simulink model "Modelo_nolineal_5GDL_2021"  (R2021b)
settings: Solver=VariableStepAuto  StartTime=0.0  StopTime=5  FixedStep=T  RelTol=1e-3
values from neighbouring files (symbols this model uses):
  g = 9.81    [Control_5GDL_2021.m]
  Ixx = pod.mass.inertia(1,1)    [Control_5GDL_2021.m]
  Iyy = pod.mass.inertia(2,2)    [Control_5GDL_2021.m]
  Izz = pod.mass.inertia(3,3)    [Control_5GDL_2021.m]
  m = pod.mass.mass    [Control_5GDL_2021.m]
  theta0 = 0    [Control_5GDL_2021.m]
  x_g = pod.geometry.x_G    [Control_5GDL_2021.m]
  x_lev = pod.geometry.x_LEV    [Control_5GDL_2021.m]
  y_lev = pod.geometry.y_LEV    [Control_5GDL_2021.m]
  z_g = pod.geometry.z_G    [Control_5GDL_2021.m]
  z_ini = z_0+z_lev    [Control_5GDL_2021.m]
undefined symbols (not defined in the file or in its folder): k1, k2, k3, k4, l1, l2, l3, p1, p2
settings Model: Creator=EDMAOR  LastModifiedBy=emate
settings SolverCC: AlgebraicLoopSolver=TrustRegion
settings DebuggingCC: SFMachineParentedDataDiag=warning
settings SFSimCC: CustomCodeUndefinedFunction=UseInterfaceOnly

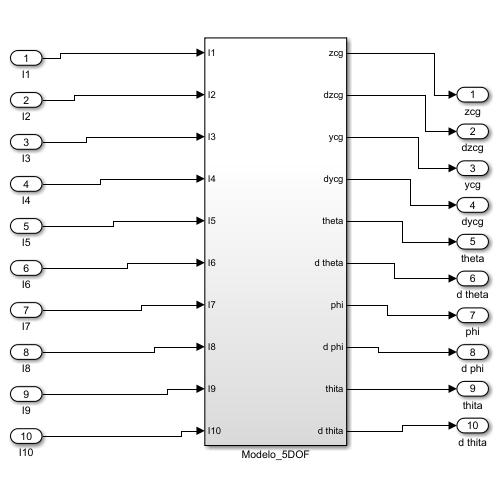
[thumbnail: Simulink's stored preview of the top-level diagram]
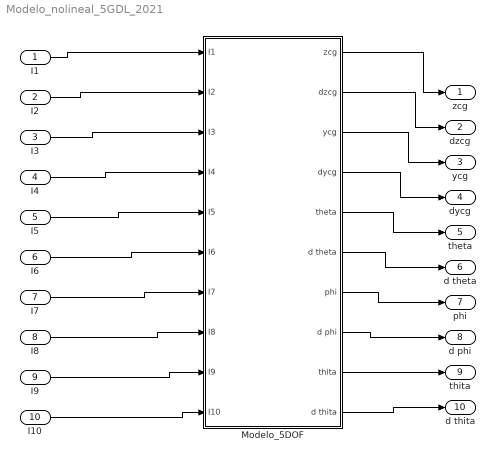
== system Modelo_nolineal_5GDL_2021 ==
  I1 : Inport
  I2 : Inport  Port=2
  I3 : Inport  Port=3
  I4 : Inport  Port=4
  I5 : Inport  Port=5
  I6 : Inport  Port=6
  I7 : Inport  Port=7
  I8 : Inport  Port=8
  I9 : Inport  Port=9
  I10 : Inport  Port=10
  Modelo_5DOF : Subsystem
  zcg : Outport  VectorParamsAs1DForOutWhenUnconnected=off
  dzcg : Outport  Port=2  VectorParamsAs1DForOutWhenUnconnected=off
  ycg : Outport  Port=3  VectorParamsAs1DForOutWhenUnconnected=off
  dycg : Outport  Port=4  VectorParamsAs1DForOutWhenUnconnected=off
  theta : Outport  Port=5  VectorParamsAs1DForOutWhenUnconnected=off
  d theta : Outport  Port=6  VectorParamsAs1DForOutWhenUnconnected=off
  phi : Outport  Port=7  VectorParamsAs1DForOutWhenUnconnected=off
  d phi : Outport  Port=8  VectorParamsAs1DForOutWhenUnconnected=off
  thita : Outport  Port=9  VectorParamsAs1DForOutWhenUnconnected=off
  d thita : Outport  Port=10  VectorParamsAs1DForOutWhenUnconnected=off
  wires:
  Modelo_5DOF/1(zcg) -> zcg/1
  I1/1 -> Modelo_5DOF/1(I1)
  I2/1 -> Modelo_5DOF/2(I2)
  I3/1 -> Modelo_5DOF/3(I3)
  I4/1 -> Modelo_5DOF/4(I4)
  I5/1 -> Modelo_5DOF/5(I5)
  I6/1 -> Modelo_5DOF/6(I6)
  Modelo_5DOF/2(dzcg) -> dzcg/1
  Modelo_5DOF/3(ycg) -> ycg/1
  Modelo_5DOF/4(dycg) -> dycg/1
  Modelo_5DOF/5(theta) -> theta/1
  Modelo_5DOF/6(d theta) -> d theta/1
  Modelo_5DOF/7(phi) -> phi/1
  Modelo_5DOF/8(d phi) -> d phi/1
  I7/1 -> Modelo_5DOF/7(I7)
  I8/1 -> Modelo_5DOF/8(I8)
  I9/1 -> Modelo_5DOF/9(I9)
  I10/1 -> Modelo_5DOF/10(I10)
  Modelo_5DOF/9(thita) -> thita/1
  Modelo_5DOF/10(d thita) -> d thita/1

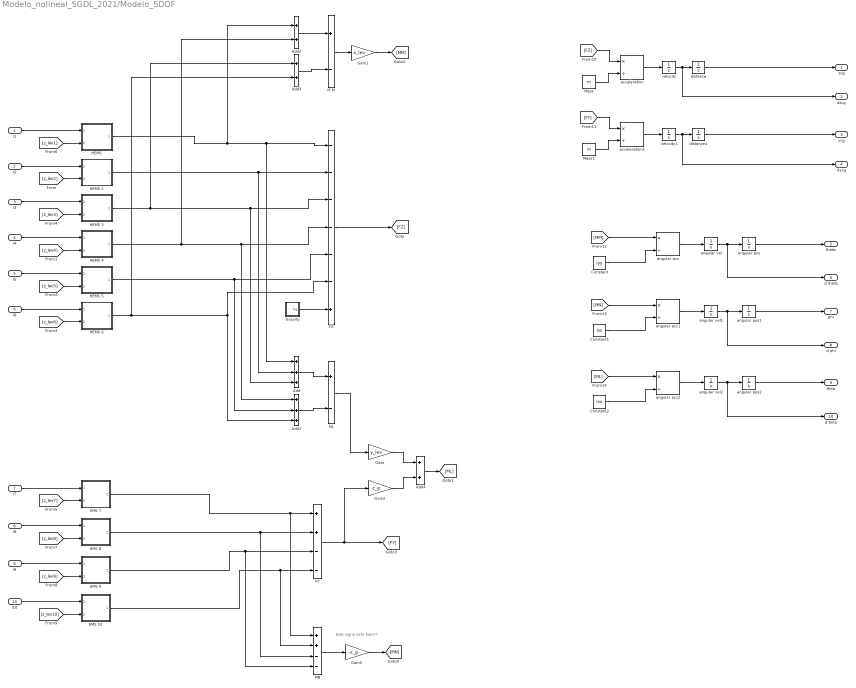
== system Modelo_nolineal_5GDL_2021/Modelo_5DOF ==
  note: Este signo esta bien??
  I1 : Inport
  I2 : Inport  Port=2
  I3 : Inport  Port=3
  I4 : Inport  Port=4
  I5 : Inport  Port=5
  I6 : Inport  Port=6
  I7 : Inport  Port=7
  I8 : Inport  Port=8
  I9 : Inport  Port=9
  I10 : Inport  Port=10
  Add : Sum  Inputs=+++
  Add1 : Sum  Inputs=+++
  Add2 : Sum
  Add3 : Sum
  Add4 : Sum
  Constant : Constant  Value=Iyy
  Constant1 : Constant  Value=Izz
  Constant2 : Constant  Value=Ixx
  EMS 10 : Subsystem
  EMS 7 : Subsystem
  EMS 8 : Subsystem
  EMS 9 : Subsystem
  FY : Sum  Inputs=++--
  FZ : Sum  Inputs=------+
  Gain : Gain  Gain=y_lev
  Gain1 : Gain  Gain=x_lev
  Gain2 : Gain  Gain=z_g
  Gain5 : Gain  Gain=-x_g
  Gravity : Subsystem
  "HEMS " : Subsystem
  HEMS 2 : Subsystem
  HEMS 3 : Subsystem
  HEMS 4 : Subsystem
  HEMS 5 : Subsystem
  HEMS 6 : Subsystem
  M M : Sum  Inputs=+-
  ML : Sum  Inputs=+-
  MN : Sum  Inputs=++--
  Mass : Constant  Value=m
  Mass1 : Constant  Value=m
  acceleration : Product  Inputs=*/
  acceleration1 : Product  Inputs=*/
  angular acc : Product  Inputs=*/
  angular acc1 : Product  Inputs=*/
  angular acc2 : Product  Inputs=*/
  angular pos : Integrator  InitialCondition=theta0
  angular pos1 : Integrator  InitialCondition=theta0
  angular pos2 : Integrator  InitialCondition=theta0
  angular vel : Integrator
  angular vel1 : Integrator
  angular vel2 : Integrator
  distance : Integrator  InitialCondition=z_ini
  distance1 : Integrator
  velocity : Integrator
  velocity1 : Integrator
  zcg : Outport  VectorParamsAs1DForOutWhenUnconnected=off
  dzcg : Outport  Port=2  VectorParamsAs1DForOutWhenUnconnected=off
  ycg : Outport  Port=3  VectorParamsAs1DForOutWhenUnconnected=off
  dycg : Outport  Port=4  VectorParamsAs1DForOutWhenUnconnected=off
  theta : Outport  Port=5  VectorParamsAs1DForOutWhenUnconnected=off
  d theta : Outport  Port=6  VectorParamsAs1DForOutWhenUnconnected=off
  phi : Outport  Port=7  VectorParamsAs1DForOutWhenUnconnected=off
  d phi : Outport  Port=8  VectorParamsAs1DForOutWhenUnconnected=off
  thita : Outport  Port=9  VectorParamsAs1DForOutWhenUnconnected=off
  d thita : Outport  Port=10  VectorParamsAs1DForOutWhenUnconnected=off
  wires:
  acceleration/1 -> velocity/1
  velocity/1 -> dzcg/1, distance/1
  distance/1 -> zcg/1
  I1/1 -> "HEMS "/1(current 1)
  I2/1 -> HEMS 2/1(current 2)
  I3/1 -> HEMS 3/1(current 3)
  "HEMS "/1(HEMS 1) -> Add/1, FZ/1, Add2/1
  HEMS 2/1(HEMS 2) -> Add/2, FZ/2
  HEMS 3/1(HEMS 3) -> Add/3, FZ/3, Add3/1
  Mass/1 -> acceleration/2
  [z_lev2] -> HEMS 2/2(distance 2)
  [z_lev3] -> HEMS 3/2(distance 3)
  [z_lev1] -> "HEMS "/2(distance 1)
  I4/1 -> HEMS 4/1(current 4)
  I5/1 -> HEMS 5/1(current 5)
  I6/1 -> HEMS 6/1(current 6)
  [z_lev4] -> HEMS 4/2(distance 4)
  [z_lev5] -> HEMS 5/2(distance 5)
  [z_lev6] -> HEMS 6/2(distance 6)
  HEMS 4/1(HEMS 4) -> Add1/1, FZ/4, Add2/2
  HEMS 5/1(HEMS 5) -> Add1/2, FZ/5
  HEMS 6/1(HEMS 6) -> Add1/3, FZ/6, Add3/2
  Gravity/1(Fg) -> FZ/7
  FZ/1 -> [FZ]
  ML/1 -> Gain/1
  Add1/1 -> ML/2
  Add/1 -> ML/1
  M M/1 -> Gain1/1
  Gain1/1 -> [MM]
  Add2/1 -> M M/1
  Add3/1 -> M M/2
  I7/1 -> EMS 7/1(current 7)
  [z_lev7] -> EMS 7/2(distance 7)
  I8/1 -> EMS 8/1(current 8)
  [z_lev8] -> EMS 8/2(distance 8)
  I9/1 -> EMS 9/1(current 9)
  [z_lev9] -> EMS 9/2(distance 9)
  I10/1 -> EMS 10/1(current 10)
  [z_lev10] -> EMS 10/2(distance 10)
  EMS 7/1(EMS 7) -> MN/1, FY/1
  EMS 8/1(EMS 8) -> MN/3, FY/2
  EMS 9/1(EMS 9) -> MN/4, FY/3
  EMS 10/1(EMS 10) -> MN/2, FY/4
  FY/1 -> [FY], Gain2/1
  Add4/1 -> [ML]
  Gain/1 -> Add4/1
  Gain2/1 -> Add4/2
  MN/1 -> Gain5/1
  Gain5/1 -> [MN]
  [FZ] -> acceleration/1
  [FY] -> acceleration1/1
  Mass1/1 -> acceleration1/2
  distance1/1 -> ycg/1
  velocity1/1 -> distance1/1, dycg/1
  acceleration1/1 -> velocity1/1
  angular vel/1 -> d theta/1, angular pos/1
  angular pos/1 -> theta/1
  angular acc/1 -> angular vel/1
  [MM] -> angular acc/1
  Constant/1 -> angular acc/2
  angular acc1/1 -> angular vel1/1
  Constant1/1 -> angular acc1/2
  angular vel1/1 -> d phi/1, angular pos1/1
  [MN] -> angular acc1/1
  angular pos1/1 -> phi/1
  angular pos2/1 -> thita/1
  [ML] -> angular acc2/1
  angular vel2/1 -> angular pos2/1, d thita/1
  Constant2/1 -> angular acc2/2
  angular acc2/1 -> angular vel2/1

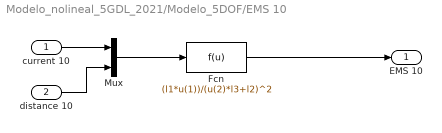
== system Modelo_nolineal_5GDL_2021/Modelo_5DOF/EMS 10 ==
  current 10 : Inport
  distance 10 : Inport  Port=2
  Fcn : Fcn  Expr=(l1*u(1))/(u(2)*l3+l2)^2
  Mux : Mux  Inputs=2
  EMS 10 : Outport  VectorParamsAs1DForOutWhenUnconnected=off
  wires:
  Fcn/1 -> EMS 10/1
  Mux/1 -> Fcn/1
  distance 10/1 -> Mux/2
  current 10/1 -> Mux/1

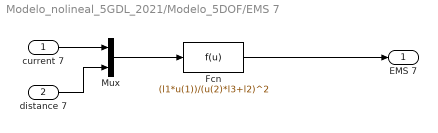
== system Modelo_nolineal_5GDL_2021/Modelo_5DOF/EMS 7 ==
  current 7 : Inport
  distance 7 : Inport  Port=2
  Fcn : Fcn  Expr=(l1*u(1))/(u(2)*l3+l2)^2
  Mux : Mux  Inputs=2
  EMS 7 : Outport  VectorParamsAs1DForOutWhenUnconnected=off
  wires:
  current 7/1 -> Mux/1
  distance 7/1 -> Mux/2
  Mux/1 -> Fcn/1
  Fcn/1 -> EMS 7/1

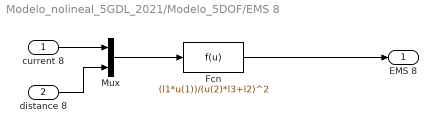
== system Modelo_nolineal_5GDL_2021/Modelo_5DOF/EMS 8 ==
  current 8 : Inport
  distance 8 : Inport  Port=2
  Fcn : Fcn  Expr=(l1*u(1))/(u(2)*l3+l2)^2
  Mux : Mux  Inputs=2
  EMS 8 : Outport  VectorParamsAs1DForOutWhenUnconnected=off
  wires:
  Fcn/1 -> EMS 8/1
  Mux/1 -> Fcn/1
  distance 8/1 -> Mux/2
  current 8/1 -> Mux/1

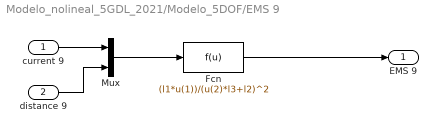
== system Modelo_nolineal_5GDL_2021/Modelo_5DOF/EMS 9 ==
  current 9 : Inport
  distance 9 : Inport  Port=2
  Fcn : Fcn  Expr=(l1*u(1))/(u(2)*l3+l2)^2
  Mux : Mux  Inputs=2
  EMS 9 : Outport  VectorParamsAs1DForOutWhenUnconnected=off
  wires:
  current 9/1 -> Mux/1
  distance 9/1 -> Mux/2
  Mux/1 -> Fcn/1
  Fcn/1 -> EMS 9/1

== system Modelo_nolineal_5GDL_2021/Modelo_5DOF/Gravity ==
  Fgrav : Subsystem
  Mass : Constant  Value=m
  gravity : Constant  Value=g
  Fg : Outport
  wires:
  Fgrav/1(Fg) -> Fg/1
  gravity/1 -> Fgrav/1(gravity)
  Mass/1 -> Fgrav/2(mass)

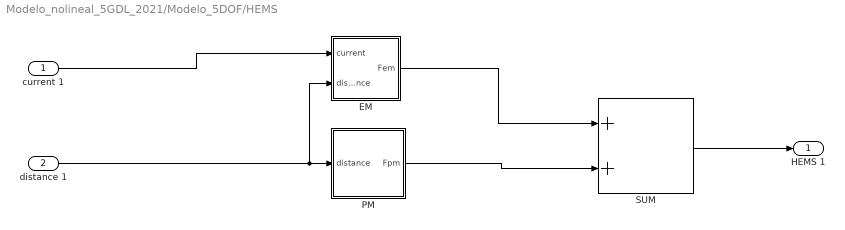
== system Modelo_nolineal_5GDL_2021/Modelo_5DOF/HEMS  ==
  current 1 : Inport
  distance 1 : Inport  Port=2
  EM : Subsystem
  PM : Subsystem
  SUM : Sum
  HEMS 1 : Outport  VectorParamsAs1DForOutWhenUnconnected=off
  wires:
  PM/1(Fpm) -> SUM/2
  distance 1/1 -> EM/2(distance), PM/1(distance)
  EM/1(Fem) -> SUM/1
  current 1/1 -> EM/1(current)
  SUM/1 -> HEMS 1/1

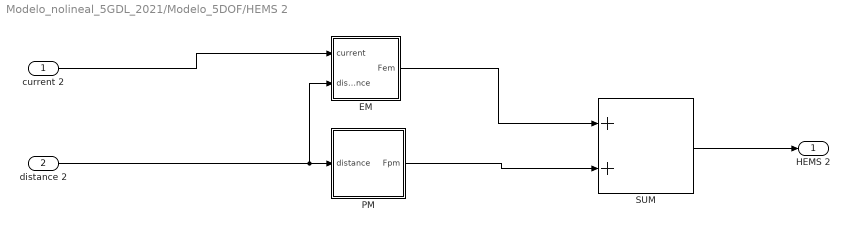
== system Modelo_nolineal_5GDL_2021/Modelo_5DOF/HEMS 2 ==
  current 2 : Inport
  distance 2 : Inport  Port=2
  EM : Subsystem
  PM : Subsystem
  SUM : Sum
  HEMS 2 : Outport  VectorParamsAs1DForOutWhenUnconnected=off
  wires:
  SUM/1 -> HEMS 2/1
  current 2/1 -> EM/1(current)
  EM/1(Fem) -> SUM/1
  distance 2/1 -> PM/1(distance), EM/2(distance)
  PM/1(Fpm) -> SUM/2

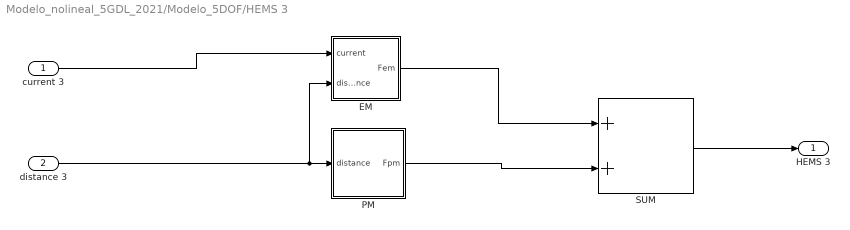
== system Modelo_nolineal_5GDL_2021/Modelo_5DOF/HEMS 3 ==
  current 3 : Inport
  distance 3 : Inport  Port=2
  EM : Subsystem
  PM : Subsystem
  SUM : Sum
  HEMS 3 : Outport  VectorParamsAs1DForOutWhenUnconnected=off
  wires:
  PM/1(Fpm) -> SUM/2
  distance 3/1 -> EM/2(distance), PM/1(distance)
  EM/1(Fem) -> SUM/1
  current 3/1 -> EM/1(current)
  SUM/1 -> HEMS 3/1

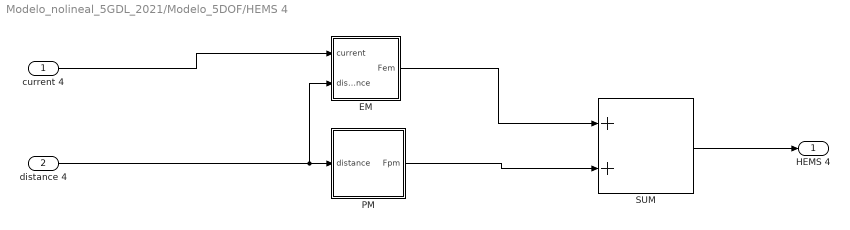
== system Modelo_nolineal_5GDL_2021/Modelo_5DOF/HEMS 4 ==
  current 4 : Inport
  distance 4 : Inport  Port=2
  EM : Subsystem
  PM : Subsystem
  SUM : Sum
  HEMS 4 : Outport  VectorParamsAs1DForOutWhenUnconnected=off
  wires:
  SUM/1 -> HEMS 4/1
  current 4/1 -> EM/1(current)
  EM/1(Fem) -> SUM/1
  distance 4/1 -> PM/1(distance), EM/2(distance)
  PM/1(Fpm) -> SUM/2

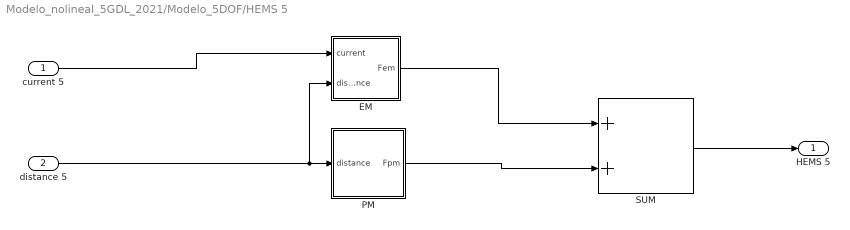
== system Modelo_nolineal_5GDL_2021/Modelo_5DOF/HEMS 5 ==
  current 5 : Inport
  distance 5 : Inport  Port=2
  EM : Subsystem
  PM : Subsystem
  SUM : Sum
  HEMS 5 : Outport  VectorParamsAs1DForOutWhenUnconnected=off
  wires:
  PM/1(Fpm) -> SUM/2
  distance 5/1 -> EM/2(distance), PM/1(distance)
  EM/1(Fem) -> SUM/1
  current 5/1 -> EM/1(current)
  SUM/1 -> HEMS 5/1

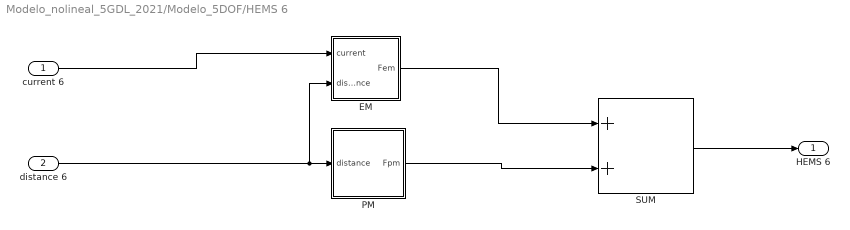
== system Modelo_nolineal_5GDL_2021/Modelo_5DOF/HEMS 6 ==
  current 6 : Inport
  distance 6 : Inport  Port=2
  EM : Subsystem
  PM : Subsystem
  SUM : Sum
  HEMS 6 : Outport  VectorParamsAs1DForOutWhenUnconnected=off
  wires:
  SUM/1 -> HEMS 6/1
  current 6/1 -> EM/1(current)
  EM/1(Fem) -> SUM/1
  distance 6/1 -> PM/1(distance), EM/2(distance)
  PM/1(Fpm) -> SUM/2

== system Modelo_nolineal_5GDL_2021/Modelo_5DOF/Gravity/Fgrav ==
  gravity : Inport
  mass : Inport  Port=2
  Product : Product
  Fg : Outport  VectorParamsAs1DForOutWhenUnconnected=off
  wires:
  Product/1 -> Fg/1
  gravity/1 -> Product/1
  mass/1 -> Product/2

== system Modelo_nolineal_5GDL_2021/Modelo_5DOF/HEMS /EM ==
  current : Inport
  distance : Inport  Port=2
  Fcn : Fcn  Expr=(k1*u(1)+k4)/(u(2)*k3-k2)^2
  Mux : Mux  Inputs=2
  Fem : Outport  VectorParamsAs1DForOutWhenUnconnected=off
  wires:
  current/1 -> Mux/1
  distance/1 -> Mux/2
  Mux/1 -> Fcn/1
  Fcn/1 -> Fem/1

== system Modelo_nolineal_5GDL_2021/Modelo_5DOF/HEMS /PM ==
  distance : Inport
  Fcn1 : Fcn  Expr=p1/(p2+u(1))^2
  Fpm : Outport  VectorParamsAs1DForOutWhenUnconnected=off
  wires:
  distance/1 -> Fcn1/1
  Fcn1/1 -> Fpm/1

== system Modelo_nolineal_5GDL_2021/Modelo_5DOF/HEMS 2/EM ==
  current : Inport
  distance : Inport  Port=2
  Fcn : Fcn  Expr=(k1*u(1)+k4)/(u(2)*k3-k2)^2
  Mux : Mux  Inputs=2
  Fem : Outport  VectorParamsAs1DForOutWhenUnconnected=off
  wires:
  Fcn/1 -> Fem/1
  Mux/1 -> Fcn/1
  distance/1 -> Mux/2
  current/1 -> Mux/1

== system Modelo_nolineal_5GDL_2021/Modelo_5DOF/HEMS 2/PM ==
  distance : Inport
  Fcn1 : Fcn  Expr=p1/(p2+u(1))^2
  Fpm : Outport  VectorParamsAs1DForOutWhenUnconnected=off
  wires:
  Fcn1/1 -> Fpm/1
  distance/1 -> Fcn1/1

== system Modelo_nolineal_5GDL_2021/Modelo_5DOF/HEMS 3/EM ==
  current : Inport
  distance : Inport  Port=2
  Fcn : Fcn  Expr=(k1*u(1)+k4)/(u(2)*k3-k2)^2
  Mux : Mux  Inputs=2
  Fem : Outport  VectorParamsAs1DForOutWhenUnconnected=off
  wires:
  current/1 -> Mux/1
  distance/1 -> Mux/2
  Mux/1 -> Fcn/1
  Fcn/1 -> Fem/1

== system Modelo_nolineal_5GDL_2021/Modelo_5DOF/HEMS 3/PM ==
  distance : Inport
  Fcn1 : Fcn  Expr=p1/(p2+u(1))^2
  Fpm : Outport  VectorParamsAs1DForOutWhenUnconnected=off
  wires:
  distance/1 -> Fcn1/1
  Fcn1/1 -> Fpm/1

== system Modelo_nolineal_5GDL_2021/Modelo_5DOF/HEMS 4/EM ==
  current : Inport
  distance : Inport  Port=2
  Fcn : Fcn  Expr=(k1*u(1)+k4)/(u(2)*k3-k2)^2
  Mux : Mux  Inputs=2
  Fem : Outport  VectorParamsAs1DForOutWhenUnconnected=off
  wires:
  Fcn/1 -> Fem/1
  Mux/1 -> Fcn/1
  distance/1 -> Mux/2
  current/1 -> Mux/1

== system Modelo_nolineal_5GDL_2021/Modelo_5DOF/HEMS 4/PM ==
  distance : Inport
  Fcn1 : Fcn  Expr=p1/(p2+u(1))^2
  Fpm : Outport  VectorParamsAs1DForOutWhenUnconnected=off
  wires:
  Fcn1/1 -> Fpm/1
  distance/1 -> Fcn1/1

== system Modelo_nolineal_5GDL_2021/Modelo_5DOF/HEMS 5/EM ==
  current : Inport
  distance : Inport  Port=2
  Fcn : Fcn  Expr=(k1*u(1)+k4)/(u(2)*k3-k2)^2
  Mux : Mux  Inputs=2
  Fem : Outport  VectorParamsAs1DForOutWhenUnconnected=off
  wires:
  current/1 -> Mux/1
  distance/1 -> Mux/2
  Mux/1 -> Fcn/1
  Fcn/1 -> Fem/1

== system Modelo_nolineal_5GDL_2021/Modelo_5DOF/HEMS 5/PM ==
  distance : Inport
  Fcn1 : Fcn  Expr=p1/(p2+u(1))^2
  Fpm : Outport  VectorParamsAs1DForOutWhenUnconnected=off
  wires:
  distance/1 -> Fcn1/1
  Fcn1/1 -> Fpm/1

== system Modelo_nolineal_5GDL_2021/Modelo_5DOF/HEMS 6/EM ==
  current : Inport
  distance : Inport  Port=2
  Fcn : Fcn  Expr=(k1*u(1)+k4)/(u(2)*k3-k2)^2
  Mux : Mux  Inputs=2
  Fem : Outport  VectorParamsAs1DForOutWhenUnconnected=off
  wires:
  Fcn/1 -> Fem/1
  Mux/1 -> Fcn/1
  distance/1 -> Mux/2
  current/1 -> Mux/1

== system Modelo_nolineal_5GDL_2021/Modelo_5DOF/HEMS 6/PM ==
  distance : Inport
  Fcn1 : Fcn  Expr=p1/(p2+u(1))^2
  Fpm : Outport  VectorParamsAs1DForOutWhenUnconnected=off
  wires:
  Fcn1/1 -> Fpm/1
  distance/1 -> Fcn1/1
